simulink model "LTI_DT_60s_sample"  (R2017a)
settings: Solver=VariableStepAuto  StartTime=0.0  StopTime=18000  RelTol=1e-3  EnableMultiTasking=on
values from neighbouring files (symbols this model uses):
  Aori = eye(no_region)+T*L*(Asys_ori + Bsys*Kv_r)*inv(L)    [Main_TreeApp_ptbMST.m]    (also in Main_TreeApp_ptbMST6.m; appTest.mat = [0.799977169598 0 0 0 0 0 0 0 0 0 0 6.32274241222e-06 ... (2; appTest6.mat = [0.799992772662 0 0 0 0 0 0 0 0 0 0 2.74335990298e-06 ... (2)
  Atree = eye(no_region)+T*L*(Asys + Bsys*Kv_r)*inv(L)    [Main_TreeApp_ptbMST.m]    (also in Main_TreeApp_ptbMST6.m; appTest.mat = [0.799977169598 0 0 0 0 0 0 0 0 0 0 6.32274241222e-06 ... (2; appTest6.mat = [0.799992772662 0 0 0 0 0 0 0 0 0 0 2.74335990298e-06 ... (2)
  disSeedArr = 1:no_region    [Main_TreeApp_ptbMST.m]    (also in Main_TreeApp_ptbMST6.m; appTest.mat = [1 2 3 4 5 6 7 8 9 10 11 12 ... (50 elements, 1x50)]; appTest6.mat = [1 2 3 4 5 6 7 8 9 10 11 12 ... (50 elements, 1x50)])
  Kv_r = [-0.00123579901274 0.000174941451611 0.00018450668775 0 0 0 0 0 0 0 0 0 ... (7400 elements, 148x50)]    [appTest.mat]    (also in appTest6.mat = [-0.00123577593006 0.000174932430697 0.000184467308148 0 0 0)
  L = [0.000430550903589 0 0 0 0 0 0 0 0 0 0 0 ... (2500 elements, 50x50)]    [appTest.mat]    (also in appTest6.mat)
  no_region = numBubbles    (= 50)    [Main_TreeApp_ptbMST.m]    (also in Main_TreeApp_ptbMST6.m; appTest.mat; appTest6.mat)
  T = 60    [Main_TreeApp_ptbMST.m]    (also in Main_TreeApp_ptbMST6.m; appTest.mat; appTest6.mat)
settings Model: Creator=yaqiz  LastModifiedBy=Yaqi
settings OptimizationCC: LifeSpan=inf
settings DebuggingCC: SFUnexpectedBacktrackingDiag=warning  SFNoUnconditionalDefaultTransitionDiag=warning  SFExecutionAtInitializationDiag=none
settings GRTTargetCC: TargetLangStandard=C89/C90 (ANSI)  GeneratePreprocessorConditionals=Disable all
settings ConfigComp: CovMetricSettings=dw  CovHtmlReporting=on  CovSaveCumulativeToWorkspaceVar=on  CovSaveSingleToWorkspaceVar=on  CovExternalEMLEnable=off

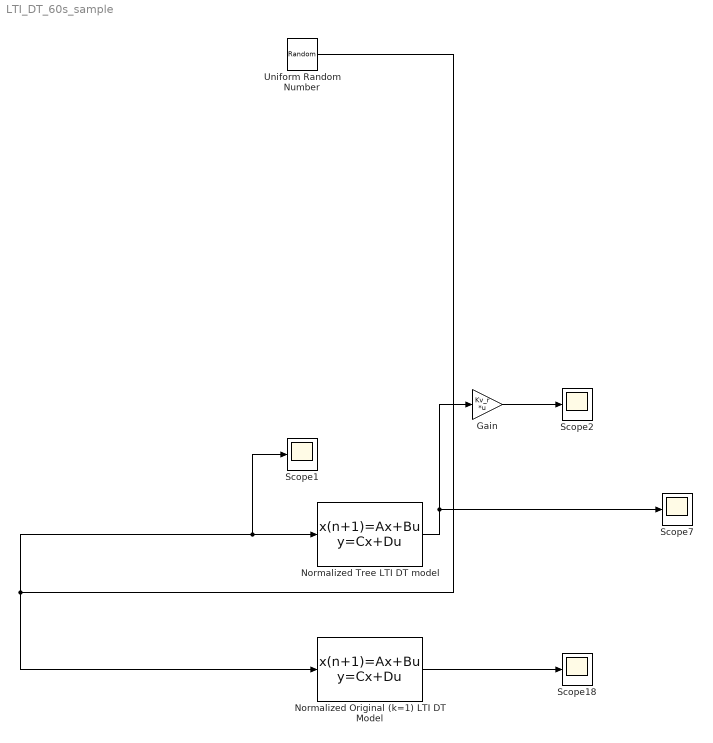
== system LTI_DT_60s_sample ==
  Gain : Gain  Gain=Kv_r  Multiplication=Matrix(K*u)
  Normalized Original (k=1) LTI DT Model : DiscreteStateSpace  A=Aori  B=L*T  C=eye(no_region)  D=zeros(no_region)  X0=zeros(no_region,1)  SampleTime=T
  Normalized Tree LTI DT model : DiscreteStateSpace  A=Atree  B=L*T  C=eye(no_region)  D=zeros(no_region)  X0=zeros(no_region,1)  SampleTime=T
  Scope{1..2,7,18} (4 alike) : Scope
  Uniform Random Number : UniformRandomNumber  Minimum=-1*ones(no_region,1)  Maximum=1*ones(no_region,1)  Seed=disSeedArr  SampleTime=T
  wires:
  Normalized Tree LTI DT model/1 -> Gain/1, Scope7/1
  Gain/1 -> Scope2/1
  Normalized Original (k=1) LTI DT Model/1 -> Scope18/1
  Uniform Random Number/1 -> Scope1/1, Normalized Tree LTI DT model/1, Normalized Original (k=1) LTI DT Model/1
